simulink library "CDS_PARTS"  (Simulink 6.5)
libraries: dac x1, cdsEpicsIn x1, cdsEpicsOut x1, cdsPPFIR x1, cdsFilt x1, cdsMatrix x1, cdsRms x1, cdsOsc x1, cdsPhase x1, cdsProduct x1, cdsRampSwitch x1, cdsRemoteIntlk x1
settings Model: Creator=aivanov  LastModifiedBy=aivanov  ExtModeAutoUpdateStatusClock=off

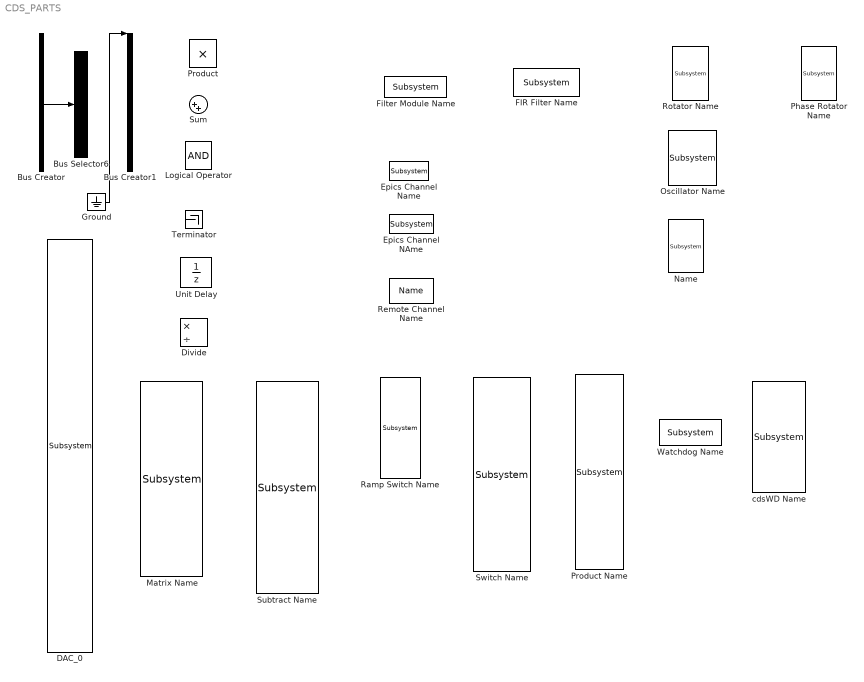
== system CDS_PARTS ==
  Bus Creator : BusCreator  Tag=adc_0  Description=ADC0  Inputs='adc_0_0','adc_0_1','adc_0_2','adc_0_3','adc_0_4','adc_0_5','adc_0_6','adc_0_7','adc_0_8','adc_0_9','adc_0_10','adc_0_11','adc_0_12','adc_0_13','adc_0_14','adc_0_15','adc_0_16','adc_0_17','adc_0_18','adc_0_19','adc_0_20','adc_0_21','adc_0_22','adc_0_23','adc_0_24','adc_0_25','adc_0_26','adc_0_27','adc_0_28','adc_0_29','adc_0_30','adc_0_31'
      settings: AttributesFormatString=%<Tag>
  Bus Creator1 : BusCreator  Description=ADC1  Inputs='adc_1_0','adc_1_1','adc_1_2','adc_1_3','adc_1_4','adc_1_5','adc_1_6','adc_1_7','adc_1_8','adc_1_9','adc_1_10','adc_1_11','adc_1_12','adc_1_13','adc_1_14','adc_1_15','adc_1_16','adc_1_17','adc_1_18','adc_1_19','adc_1_20','adc_1_21','adc_1_22','adc_1_23','adc_1_24','adc_1_25','adc_1_26','adc_1_27','adc_1_28','adc_1_29','adc_1_30','adc_1_31'
      settings: AttributesFormatString=%<Description>
  Bus Selector6 : BusSelector  Description=ADC Selector  OutputSignals=adc_0_0,adc_0_1
      settings: AttributesFormatString=%<Description>
  DAC_0 : dac/Subsystem  Description=DAC  SystemSampleTime=-1
      settings: AttributesFormatString=%<Description>
  Divide : Product  Inputs=*/  OutScaling=2^-10
  Epics Channel NAme : cdsEpicsIn/Subsystem  Tag=cdsEpicsInput  Description=|  SystemSampleTime=-1
      | Purpose:                                                                              
      | Create an EPICS input channel connection to the FE realtime controls.                 
      |                                                                                       
      | Operation:                                                                            
      | Outputs value from an EPICS ai record. Value is floating point with a precision of 3..
      |                                                                                       
      | Usage:                                                                                
      | Name the part with the desired EPICS channel name.
      settings: AttributesFormatString=%<Tag>
  Epics Channel Name : cdsEpicsOut/Subsystem  Tag=cdsEpicsOutput  Description=|  SystemSampleTime=-1
      | Purpose:                                          
      | Output a FE signal to an EPICS channel.           
      |                                                   
      | Operation:                                        
      | Takes input value and passes it to EPICS record.  
      |                                                   
      | Usage:                                            
      | Name the part with the desired EPICS rrecord name.
      settings: AttributesFormatString=%<Tag>
  FIR Filter Name : cdsPPFIR/Subsystem  Tag=cdsPPFIR  Description=|  SystemSampleTime=-1
      | Purpose:                                                                                                    
      | Provide a Polyphase FIR filter algorithm. This part is typically only used in HEPI or other seismic systems.
      settings: AttributesFormatString=%<Tag>
  Filter Module Name : cdsFilt/Subsystem  Tag=cdsFilt  Description=|  SystemSampleTime=-1
      | Purpose:                                                                                                                                                                                                                                  
      | Standard CDS IIR filter module.                                                                                                                                                                                                           
      |                                                                                                                                                                                                                                           
      | Operation:                                                                                                                                                                                                                                
      | Consists of 10 second order section IIR filters, plus a ramped gain stage. In FE code, also provides pre-defined test points and excitation channel inputs. The filter coefficients are defined in the LIGO system using the 'foton' tool.
      |                                                                                                                                                                                                                                           
      | Usage:                                                                                                                                                                                                                                    
      | Name the part with the desired filter module name.
      settings: AttributesFormatString=%<Tag>
  Ground : Ground
  Logical Operator : Logic  AllPortsSameDT=off  OutDataTypeMode=Boolean
  Matrix Name : cdsMatrix/Subsystem  Tag=Matrix  Description=|  SystemSampleTime=-1
      | Purpose:                                                                 
      | Provide a matrix multiplication function for up to 8 input and 8 outputs.
      settings: AttributesFormatString=%<Tag>
  Name : cdsRms/Subsystem  Tag=cdsRms  Description=|  SystemSampleTime=-1
      | Purpose:
      | Calculate an RMS based on the input signal.
      settings: AttributesFormatString=%<Tag>
  Oscillator Name : cdsOsc/Subsystem  Tag=cdsOsc  Description=Oscillator  SystemSampleTime=-1
      settings: AttributesFormatString=%<Tag>
  Phase Rotator Name : cdsPhase/Subsystem  Tag=cdsPhase  Description=Phase Rotator  SystemSampleTime=-1
      settings: AttributesFormatString=%<Tag>
  Product : Product  RndMeth=Zero
  Product Name : cdsProduct/Subsystem  Tag=cdsProduct  Description=|  SystemSampleTime=-1
      | Purpose:                                                                                                                                                                      
      | Multiply 8 inputs by a common gain factor.                                                                                                                                    
      |                                                                                                                                                                               
      | Operation:                                                                                                                                                                    
      | Generates two epics records: partName and partName_TRAMP. All eight inputs are multiplied by the EPICS partName input, ramped over a duration (in seconds) of the TRAMP input.
      settings: AttributesFormatString=%<Tag>
  Ramp Switch Name : cdsRampSwitch/Subsystem  Tag=cdsRampSwitch  Description=Ramp Switch  SystemSampleTime=-1
      settings: AttributesFormatString=%<Tag>
  Remote Channel Name : cdsRemoteIntlk/Name  Tag=cdsRemoteIntlk  Description=|  SystemSampleTime=-1
      | Purpose:                                                                                                                                                                                                                                                                            
      | Used to turn off a switch in another subsystem using EPICS channel access. Typically, this is used as a remote interlock function.                                                                                                                                                  
      |                                                                                                                                                                                                                                                                                     
      | Operation:                                                                                                                                                                                                                                                                          
      | If input is zero, sends a zero to the specified EPICS channel name. Any other input value results in a NOOP. Input must be an integer.                                                                                                                                              
      |                                                                                                                                                                                                                                                                                     
      | Usage: Give the name of the EPICS channel to be written to, including the subsystem. For example: SEI-HMY_ACT_SW. This function will also produce a local EPICS variable for monitoring. For example, the above would result in a local EPICS variable of IFO:SUBSYS-SEI_HMY_ACT_SW.
      settings: AttributesFormatString=%<Tag>
  Rotator Name : cdsWfsPhase/Subsystem  Tag=cdsWfsPhase  Description=WFS Phase Rotator  SystemSampleTime=-1
      settings: AttributesFormatString=%<Tag>
  Subtract Name : cdsSubtract8/Subsystem  Tag=cdsSubtract8  Description=|  SystemSampleTime=-1
      | Purpose:
      | Subtract pairs of 16 inputs.
      settings: AttributesFormatString=%<Tag>
  Sum : Sum  Inputs=|++
  Switch Name : cdsSwitch1/Subsystem  Tag=cdsSwitch1  Description=Switch  SystemSampleTime=-1
      settings: AttributesFormatString=%<Tag>
  Terminator : Terminator
  Unit Delay : UnitDelay
  Watchdog Name : cdsSusWd/Subsystem  Tag=cdsSusWd  Description=Sus Watchdog  SystemSampleTime=-1
      settings: AttributesFormatString=%<Tag>
  cdsWD Name : cdsWD/Subsystem  Description=cdsWD  SystemSampleTime=-1
      settings: AttributesFormatString=%<Description>
  wires:
  Bus Creator/1 -> Bus Selector6/1
  Ground/1 -> Bus Creator1/1
